simulink model "one_sub_model"  (Simulink 8.4)
settings: Solver=FixedStepDiscrete  StartTime=0.0  StopTime="                                                                                 300"  FixedStep=1/256  RelTol=1e-3
undefined symbols (not defined in the file): currentCFG_one_sub_model_UB, UB
libraries: gRTanalyze x3, Tools x1, gUSBamplib x1
settings Model: Creator=2110973l  LastModifiedBy=2110973l
settings DataIOCC: SignalLoggingSaveFormat=Dataset
settings OptimizationCC: ExpressionDepthLimit=128
settings DebuggingCC: UnderspecifiedInitializationDetection=Simplified  MergeDetectMultiDrivingBlocksExec=error  FcnCallInpInsideContextMsg=EnableAllAsError  StateNameClashWarn=none
settings GRTTargetCC: CombineOutputUpdateFcns=on  GRTInterface=off

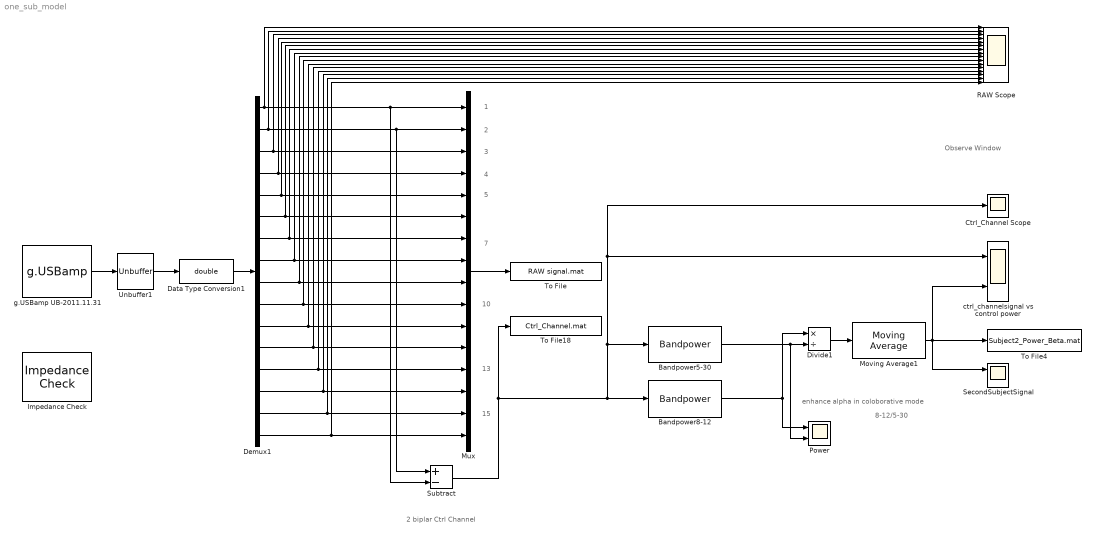
== system one_sub_model ==
  note: 13
  note: 15
  note: 4
  note: 3
  note: 7
  note: 10
  note: 5
  note: 2
  note: 1
  note: Observe Window
  note: 2 biplar Ctrl Channel
  note: enhance alpha in coloborative mode
  note: 8-12/5-30
  Bandpower5-30 : gRTanalyze/Bandpower  Order=5  LowerFreq=5  UpperFreq=30  WindowLength=128
  Bandpower8-12 : gRTanalyze/Bandpower  Order=5  LowerFreq=8  UpperFreq=12  WindowLength=128
  Ctrl_Channel Scope : Scope
      settings: YMin=-100  YMax=100
  Data Type Conversion1 : DataTypeConversion  OutDataTypeStr=double
  Demux1 : Demux  Outputs=16
  Divide1 : Product  Inputs=*/
  Impedance Check : Tools/Impedance Check  SystemSampleTime=-1
  Moving Average1 : gRTanalyze/Moving Average  windowSize=256
  Mux : Mux  Inputs=16
  Power : Scope  NumInputPorts=2
      settings: YMin=0~0  YMax=1200~1200  SaveName=ScopeData5
  RAW Scope : Scope  NumInputPorts=16
      settings: YMin=-50~-50~-50~-50~-50~-50~-50~-50~-50~-50~-50~-50~-100~-50~-100~-100  YMax=50~50~50~50~50~50~50~50~50~50~50~50~100~50~100~100
  SecondSubjectSignal : Scope  NumInputPorts=2
      settings: YMin=1.014~-1  YMax=1.032~1  SaveName=ScopeData3
  Subtract : Sum  Inputs=+-
  To File : ToFile  Filename=RAW signal.mat  MatrixName=AllChannel
  To File18 : ToFile  Filename=Ctrl_Channel.mat  MatrixName=Ctrl_Channel
  To File4 : ToFile  Filename=Subject2_Power_Beta.mat  MatrixName=Subject2_Power_Beta
  Unbuffer1 : Unbuffer  SampleBasedProcessing=Same as frame based
  ctrl_channelsignal vs control power : Scope  NumInputPorts=2
      settings: YMin=-100~0  YMax=100~20  SaveName=ScopeData7
  g.USBamp UB-2011.11.31 : gUSBamplib/g.USBamp  cfg=currentCFG_one_sub_model_UB-2011.11.31.cfg  snr=UB-2011.11.31
  wires:
  Bandpower8-12/1 -> Divide1/1, Power/1
  Bandpower5-30/1 -> Divide1/2, Power/2
  Moving Average1/1 -> To File4/1, ctrl_channelsignal vs control power/2, SecondSubjectSignal/1
  Divide1/1 -> Moving Average1/1
  g.USBamp UB-2011.11.31/1 -> Unbuffer1/1
  Unbuffer1/1 -> Data Type Conversion1/1
  Data Type Conversion1/1 -> Demux1/1
  Demux1/11 -> RAW Scope/11, Mux/11
  Demux1/13 -> RAW Scope/13, Mux/13
  Demux1/15 -> RAW Scope/15, Mux/15
  Demux1/1 -> Subtract/2, Mux/1, RAW Scope/1
  Demux1/7 -> RAW Scope/7, Mux/7
  Demux1/9 -> RAW Scope/9, Mux/9
  Subtract/1 -> Bandpower5-30/1, Ctrl_Channel Scope/1, ctrl_channelsignal vs control power/1, Bandpower8-12/1, To File18/1
  Demux1/2 -> Subtract/1, Mux/2, RAW Scope/2
  Demux1/4 -> Mux/4, RAW Scope/4
  Demux1/6 -> RAW Scope/6, Mux/6
  Demux1/8 -> RAW Scope/8, Mux/8
  Demux1/12 -> RAW Scope/12, Mux/12
  Demux1/14 -> RAW Scope/14, Mux/14
  Demux1/16 -> RAW Scope/16, Mux/16
  Demux1/5 -> RAW Scope/5, Mux/5
  Demux1/3 -> Mux/3, RAW Scope/3
  Demux1/10 -> RAW Scope/10, Mux/10
  Mux/1 -> To File/1
